simulink model "ModelMedusa"  (R2022b)
settings: Solver=FixedStepDiscrete  StartTime=0.0  StopTime=1  RelTol=1e-3  EnableMultiTasking=on
InitFcn:
  | % Initialize model
  | run(['ModelInit.m']);
  | 
  | % load library data
  | GainLibrary_data;
StartFcn:
  | % make sure all the simulated RTC requests are found
  | %RTC_SIM_OBJ.ValidateREQs();
model workspace (MAT data in the model file):
  PreampVolumeTable_Idx : Simulink.Signal (value not decoded)
  Range : Simulink.Signal (value not decoded)
  Table_Idx : Simulink.Signal (value not decoded)
undefined symbols (not defined in the file): Config, IFIR, Ifir, MedusaConfig, numAudioIn, Row, sys_defs, VLSConfig
libraries: TuneVar x16, FeaturePath x15, MedusaDelays x9, RTC x5, TOP x5, SampleRateConverter x4, dspindex x3, EdgePorts x2, MedusaCaeEnable x2, FIREven x2, VLSGains x2, dspsrcs4 x2
(part 2 of 2)

== system ModelMedusa/PreAmp/DecRate/Medusa5H1/MedusaHoligram/Medusa5H1 Part 4/On ==
  note: To fix the Headrest EQ link, FIR generic filter needs to work for multiple instances.
  HeadrestPremixOut : Inport
  NonHeadrestPremixOut : Inport  Port=2  OutDataTypeStr=single
  FRMixerOut : Inport  Port=3  OutDataTypeStr=single
  Action Port : ActionPort  ActionPortLabel=if(u1 > 0)
  DR Mix Matrix with Hybrid Holigram EQ : MedusaDRHoligramEQ/DR Holigram EQ  configStruct=config.HoligramEQConfig
  FR IIR Holigram EQ : MedusaFRHoligramEQ/FR Holigram EQ  configStruct=config.HoligramEQConfig
  Headrest Comp EQ : Subsystem  AncestorBlock=HeadrestCompEQ/Headrest Comp EQ  mask{configStruct=vlsConfigStruct.HeadrestCompEQConfig}
      mask prompts: configStruct "Config struct name:"
      mask init:
      | % Get block parameters from configStruct
      | fixedDelayLength = configStruct.fixedDelayLength;
      | IIR = configStruct.DRIIR;
      | variantFIR = configStruct.variantFIR;
      | variantIIR = configStruct.variantIIR;
      | firLength = configStruct.firLength;
      | frameSize = configStruct.frameSize;
      | numEQlink = configStruct.numEQlink;
      | numInput = configStruct.numInput;
      | 
      | % Get block default values
      | firCoeffsDefault = configStruct.firCoeffsDefault;
      | 
      | % Set implementation type for FIR
      | firBlockPath = MaskUtil.SubBlockName(gcbh, 'FIR');
      | firBlockHandle = getSimulinkBlockHandle(firBlockPath);
      | if -1 ~= firBlockHandle
      |     set_param(firBlockHandle, 'variantSelect', variantFIR);
      |     if variantFIR == 1 % Set two extras block params for Accel implementation
      |         set_param(firBlockHandle, 'numIn', num2str(numInput));
      |         set_param(firBlockHandle, 'frameSize', num2str(frameSize));
      |     end
      | end
      | 
      | iirBlockPath = MaskUtil.SubBlockName(gcbh, 'IIR');
      | iirBlockHandle = getSimulinkBlockHandle(iirBlockPath);
      | if -1 ~= iirBlockHandle
      |     set_param(iirBlockHandle, 'variantSelect', variantIIR);
      |     if variantIIR == 1 % Set two extras block params for Accel implementation
      |         set_param(iirBlockHandle, 'numChannels', num2str(numEQlink));
      |         set_param(iirBlockHandle, 'frameSize', num2str(frameSize));
      |     end
      | end
      settings: LibrarySourceBlock=HeadrestCompEQ/Headrest Comp EQ
  Matrix Concatenate : Concatenate  Mode=Multidimensional array  ConcatenateDimension=2
  DROut : Outport  VectorParamsAs1DForOutWhenUnconnected=off
  FROut : Outport  Port=2  VectorParamsAs1DForOutWhenUnconnected=off
  wires:
  FR IIR Holigram EQ/1 -> FROut/1
  Matrix Concatenate/1 -> DROut/1
  Headrest Comp EQ/1(Components Out) -> Matrix Concatenate/2
  DR Mix Matrix with Hybrid Holigram EQ/1 -> Matrix Concatenate/1
  FRMixerOut/1 -> FR IIR Holigram EQ/1
  NonHeadrestPremixOut/1 -> DR Mix Matrix with Hybrid Holigram EQ/1
  HeadrestPremixOut/1 -> Headrest Comp EQ/1(Components In)

== system ModelMedusa/PreAmp/DecRate/Medusa5H1/MedusaHoligram/Medusa5H1 Part 5/Speaker Delay Tune ==
  Output Delay Translation with Headrest : MedusaDelays/HeadrestOutputDelayTranslation  Config=[]
  TOP3 : TOP/TOP  TriggerInit=[645 305 895 365]  TopName=FRSpeakerDelay  DataType=int32  BankNumber=0  PreOverlay=false  PostOverlay=false  Role=Automatic
      settings: SourceProductName=Bose Talaria
  TOP5 : TOP/TOP  TriggerInit=[645 155 895 215]  TopName=DRSpeakerDelay  DataType=int32  BankNumber=0  PreOverlay=false  PostOverlay=false  Role=Automatic
      settings: SourceProductName=Bose Talaria
  Tune Variable : TuneVar/TuneVar  TuneName=HeadrestDrvSpeakerDelaySamples  SpecifyMaxSize=off  VariableDim=1 (Row)  MaxSize=[1 1]  TunabilityNumber=1  MinValue=[]  MaxValue=[]  TriggerInit=[20 195 245 245]  MaskValue=[0]
      settings: SourceProductName=Bose Talaria
  Tune Variable1 : TuneVar/TuneVar  TuneName=NonHeadrestSpeakerDelaySamples  SpecifyMaxSize=off  VariableDim=1 (Row)  MaxSize=[1 1]  TunabilityNumber=1  MinValue=[]  MaxValue=[]  TriggerInit=[20 120 245 170]  MaskValue=HRDelayConfig.DRNonHRDelay
      settings: SourceProductName=Bose Talaria
  Tune Variable4 : TuneVar/TuneVar  TuneName=HeadrestPaxSpeakerDelaySamples  SpecifyMaxSize=off  VariableDim=1 (Row)  MaxSize=[1 1]  TunabilityNumber=1  MinValue=[]  MaxValue=[]  TriggerInit=[20 270 245 320]  MaskValue=[0]
      settings: SourceProductName=Bose Talaria
  Tune Variable5 : TuneVar/TuneVar  TuneName=FRHoligramDelaySamples  SpecifyMaxSize=off  VariableDim=1 (Row)  MaxSize=[]  TunabilityNumber=1  MinValue=[]  MaxValue=[]  TriggerInit=[20 345 245 395]  MaskValue=HRDelayConfig.FRSpkrDelay
      settings: SourceProductName=Bose Talaria
  DRSpeakerDelay : Outport
  FRSpeakerDelay : Outport  Port=2
  wires:
  Output Delay Translation with Headrest/2 -> TOP3/1
  Output Delay Translation with Headrest/1 -> TOP5/1
  Tune Variable5/1 -> Output Delay Translation with Headrest/4  "FRHoligramDelaySamples"
  Tune Variable4/1 -> Output Delay Translation with Headrest/3  "HeadrestPaxSpeakerDelaySamples"
  Tune Variable/1 -> Output Delay Translation with Headrest/2  "HeadrestDrvSpeakerDelaySamples"
  Tune Variable1/1 -> Output Delay Translation with Headrest/1  "NonHeadrestSpeakerDelaySamples"
  TOP3/1 -> FRSpeakerDelay/1  "FRSpeakerDelay"
  TOP5/1 -> DRSpeakerDelay/1  "DRSpeakerDelay"

== system ModelMedusa/PreAmp/DecRate/Medusa5H1/MedusaHoligram/Medusa5H1 Part 1/CAE Treble Boost/Audio Passthrough ==
  AudioIn : Inport
  Constant : Constant  Value=0  OutDataTypeStr=int32  SampleTime=-1
  Constant3 : Constant  Value=0  OutDataTypeStr=int32  SampleTime=-1
  Target StateVar : StateVar/TargetStateVar  TriggerInit=[235 166 375 234]  TspName=DummyState  StateName=DummyState  UseSameName=on  IfdefMacro=[]
      settings: SourceProductName=Bose Talaria
  Terminator : Terminator
  TuneTOP : TuneVar/TuneTOP  TriggerInit=[50 262 220 318]  TopName=DummyTune  TuneName=DummyTune  DataType=single  TunabilityNumber=1  MinValue=[]  MaxValue=[]  BankNumber=0  PreOverlay=false  PostOverlay=false  UseSameName=on  MaskValue=[1]
      settings: SourceProductName=Bose Talaria
  Out : Outport
  CAEEnable : Outport  Port=2
  wires:
  Constant3/1 -> CAEEnable/1
  Constant/1 -> Target StateVar/1
  TuneTOP/1 -> Terminator/1
  AudioIn/1 -> Out/1

== system ModelMedusa/PreAmp/DecRate/Medusa5H1/MedusaHoligram/Medusa5H1 Part 1/CAE Treble Boost/CAE Treble Boost  ==
  AudioIn : Inport
  CAE Enable : MedusaCaeEnable/MedusaCaeEnable  Config=Config.CaeEnable  MaskMessageName=CAEEnable
  Treble Boost : TrebleBoost/TrebleBoostStereo  Config=Config.TrebleBoost
  Tune Variable4 : TuneVar/TuneVar  Description=|  TuneName=SurroundOn  SpecifyMaxSize=off  VariableDim=1 (Row)  MaxSize=[1 1]  TunabilityNumber=1  MinValue=[]  MaxValue=[]  TriggerInit=[-50 35 120 85]  MaskValue=2
      | General surround control parameter
      | STEREO_MODE = 0
      | SURROUND_PASSTHRU_MODE = 1
      | MEDUSA_2_CHANNEL_MODE = 2
      | MEDUSA_5_1_MODE = 3
      settings: SourceProductName=Bose Talaria
  Out : Outport
  CAEEnable : Outport  Port=2
  wires:
  Treble Boost/1 -> Out/1
  AudioIn/1 -> Treble Boost/1
  Tune Variable4/1 -> Treble Boost/2  "SurroundOn"
  CAE Enable/1 -> CAEEnable/1, Treble Boost/3

== system ModelMedusa/PreAmp/DecRate/Medusa5H1/MedusaHoligram/Medusa5H1 Part 1/Medusa Band Split Stereo/Interpolated Filter ==
  AudioIn : Inport
  Data Store Memory : DataStoreMemory  DataStoreName=states  ReadBeforeWriteMsg=warning  WriteAfterWriteMsg=warning  WriteAfterReadMsg=warning  InitialValue=zeros(size(coeffsFlip,1)*I,numChannels)  ShowAdditionalParam=off  OutDataTypeStr=single
  ifir : MATLAB Function  TreatAsAtomicUnit=on
  AudioOut : Outport  VectorParamsAs1DForOutWhenUnconnected=off
  wires:
  ifir/1(audioOut) -> AudioOut/1
  AudioIn/1 -> ifir/1(audioIn)

== system ModelMedusa/PreAmp/DecRate/Medusa5H1/MedusaHoligram/Medusa5H1 Part 3/On/Delay Tuning ==
  Delay Translation : MedusaDelays/MedusaAlignmentDelayTranslation  Config=Config.AlignmentDelayTranslation
  Tune Variable : TuneVar/TuneVar  TuneName=WiggleFilterDelayDecRateSamples1  SpecifyMaxSize=off  VariableDim=1 (Row)  MaxSize=[1 1]  TunabilityNumber=1  MinValue=[]  MaxValue=[]  TriggerInit=[-115 25 55 75]  MaskValue=Config.AlignmentDelayTranslation.DefaultTuning.DeciRateWiggleDelay
      settings: SourceProductName=Bose Talaria
  Tune Variable1 : TuneVar/TuneVar  TuneName=NEARWiggleFilterDelayDecRateSamples1  SpecifyMaxSize=off  VariableDim=1 (Row)  MaxSize=[1 1]  TunabilityNumber=1  MinValue=[]  MaxValue=[]  TriggerInit=[-115 87 55 133]  MaskValue=Config.AlignmentDelayTranslation.DefaultTuning.DeciRateNearWiggleDelay
      settings: SourceProductName=Bose Talaria
  Out1 : Outport
  Out2 : Outport  Port=2
  Out3 : Outport  Port=3
  wires:
  Tune Variable1/1 -> Delay Translation/2  "NEARWiggleFilterDelayDecRateSamples1"
  Delay Translation/3 -> Out3/1
  Delay Translation/1 -> Out1/1
  Delay Translation/2 -> Out2/1
  Tune Variable/1 -> Delay Translation/1  "WiggleFilterDelayDecRateSamples1"

== system ModelMedusa/PreAmp/DecRate/Medusa5H1/MedusaHoligram/Medusa5H1 Part 3/On/Expand Tail Components ==
  Tail Comps : Inport
  Constant : Constant  Value=[0 1 2 3]  OutDataTypeStr=single  SampleTime=-1
  Tail Component EQ : PooliirLib/PooliirwithNonTrivialTranslations  maxNumStages=tailCompEQ.maxNumStages  numStages=tailCompEQ.numStages  sosCoefficients=tailCompEQ.coeffs  FeatureName=tailCompEQ
  TuneTOP : TuneVar/TuneTOP  TriggerInit=[265 167 435 223]  TopName=WiggleFilter  TuneName=WiggleFilter  DataType=single  TunabilityNumber=1  MinValue=[]  MaxValue=[]  BankNumber=0  PreOverlay=false  PostOverlay=false  UseSameName=on  MaskValue=config.wiggleFilterDefault
      settings: SourceProductName=Bose Talaria
  Wiggle Filters : FIREven/FIR Even  variantSelect=Hexagon
      settings: SourceProductName=Bose Blocklib
  Wiggle Comps : Outport  VectorParamsAs1DForOutWhenUnconnected=off
  wires:
  Tail Comps/1 -> Wiggle Filters/1  "Ltail, Rtail, Ltail, Rtail"
  Tail Component EQ/1 -> Wiggle Comps/1
  Constant/1 -> Wiggle Filters/3
  TuneTOP/1 -> [wiggleFilter]
  Wiggle Filters/1 -> Tail Component EQ/1  "Lftail, Rftail, Lrtail, Rrtail"
  [wiggleFilter] -> Wiggle Filters/2

== system ModelMedusa/PreAmp/DecRate/Medusa5H1/MedusaHoligram/Medusa5H1 Part 3/On/Full-rate Mixer ==
  Upmix In : Inport
  CAE Control : Inport  Port=2
  Full-Rate Mixer with CAE & Fade Ramper : MedusaFullRateMixer/Full-Rate Mixer with CAE & Fade Ramper  MedusaFRMConfig=config.FRMConfig  MedusaFRMTune=config.FRMTune
  Out1 : Outport
  tag scope: NTFDone2=global
  wires:
  CAE Control/1 -> Full-Rate Mixer with CAE & Fade Ramper/9
  [SLC_On] -> Full-Rate Mixer with CAE & Fade Ramper/5
  [NTFCheck2] -> Full-Rate Mixer with CAE & Fade Ramper/8
  [BackFadeGain] -> Full-Rate Mixer with CAE & Fade Ramper/3
  [SurroundInfo] -> Full-Rate Mixer with CAE & Fade Ramper/7
  [SLCTrigger2] -> Full-Rate Mixer with CAE & Fade Ramper/6
  Full-Rate Mixer with CAE & Fade Ramper/2 -> [NTFDone2]
  [SLCReset2] -> Full-Rate Mixer with CAE & Fade Ramper/4
  [FrontFadeGain] -> Full-Rate Mixer with CAE & Fade Ramper/2
  Full-Rate Mixer with CAE & Fade Ramper/1 -> Out1/1
  Upmix In/1 -> Full-Rate Mixer with CAE & Fade Ramper/1

== system ModelMedusa/PreAmp/DecRate/Medusa5H1/MedusaHoligram/Medusa5H1 Part 3/On/Premix ==
  Bass In : Inport
  Upmix In : Inport  Port=2
  Wiggle In : Inport  Port=3
  CAE Control : Inport  Port=4
  Premix with Mono-Surround & CAE with Fade Ramper : MedusaPremix/PremixWithMonoSurroundAndCaeWithFadeRamper  MedusaPremixConfig=config.PremixConfig  MedusaPremixTune=config.PremixTune  MSConfig=config.MSConfig
  Out1 : Outport
  tag scope: NTFDone1=global
  wires:
  [SLC_On] -> Premix with Mono-Surround & CAE with Fade Ramper/7
  CAE Control/1 -> Premix with Mono-Surround & CAE with Fade Ramper/11
  Premix with Mono-Surround & CAE with Fade Ramper/1 -> Out1/1
  Premix with Mono-Surround & CAE with Fade Ramper/2 -> [NTFDone1]
  Upmix In/1 -> Premix with Mono-Surround & CAE with Fade Ramper/2
  Wiggle In/1 -> Premix with Mono-Surround & CAE with Fade Ramper/3
  [BackFadeGain] -> Premix with Mono-Surround & CAE with Fade Ramper/5
  [NTFCheck1] -> Premix with Mono-Surround & CAE with Fade Ramper/10
  [SLCReset1] -> Premix with Mono-Surround & CAE with Fade Ramper/6
  [SLCTrigger1] -> Premix with Mono-Surround & CAE with Fade Ramper/8
  [FrontFadeGain] -> Premix with Mono-Surround & CAE with Fade Ramper/4
  [SurroundInfo] -> Premix with Mono-Surround & CAE with Fade Ramper/9
  Bass In/1 -> Premix with Mono-Surround & CAE with Fade Ramper/1

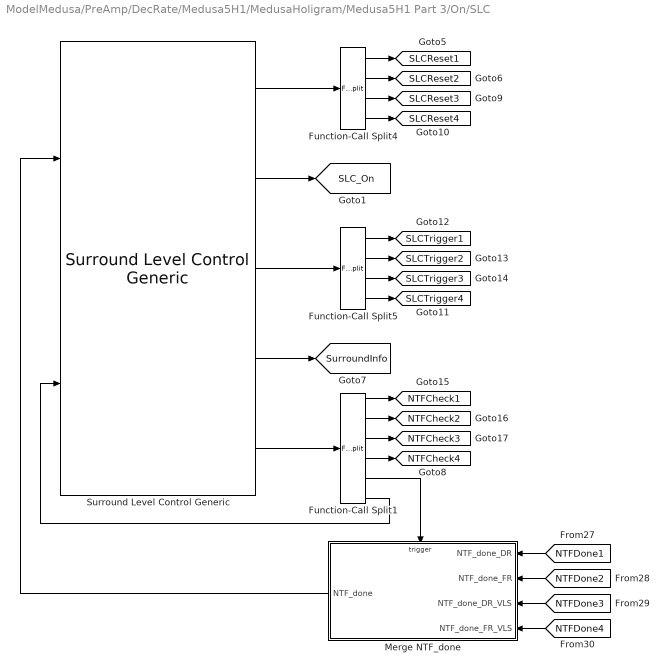
== system ModelMedusa/PreAmp/DecRate/Medusa5H1/MedusaHoligram/Medusa5H1 Part 3/On/SLC ==
  Function-Call Split1 : FunctionCallSplit  IconShape=distinctive  NumOutputPorts=6  OutputPortLayout=default
  Function-Call Split4 : FunctionCallSplit  IconShape=distinctive  NumOutputPorts=4  OutputPortLayout=default
  Function-Call Split5 : FunctionCallSplit  IconShape=distinctive  NumOutputPorts=4  OutputPortLayout=default
  Merge NTF_done : Subsystem
  Surround Level Control Generic : MedusaSurroundLevelControl/Surround Level Control Generic  SurroundConfig=config.SurroundConfig
  tag scope: NTFCheck1=global, NTFCheck2=global, NTFCheck3=global, NTFCheck4=global, SLCReset1=global, SLCReset2=global, SLCReset3=global, SLCReset4=global, SLCTrigger1=global, SLCTrigger2=global, SLCTrigger3=global, SLCTrigger4=global, SLC_On=global, SurroundInfo=global
  wires:
  Function-Call Split1/6 -> Surround Level Control Generic/2
  Surround Level Control Generic/2 -> [SLC_On]
  Surround Level Control Generic/5 -> Function-Call Split1/1
  Merge NTF_done/1(NTF_done) -> Surround Level Control Generic/1
  [NTFDone3] -> Merge NTF_done/3(NTF_done_DR_VLS)
  Function-Call Split4/4 -> [SLCReset4]
  Function-Call Split5/3 -> [SLCTrigger3]
  Function-Call Split5/1 -> [SLCTrigger1]
  Surround Level Control Generic/3 -> Function-Call Split5/1
  Surround Level Control Generic/4 -> [SurroundInfo]
  Function-Call Split4/1 -> [SLCReset1]
  Function-Call Split5/4 -> [SLCTrigger4]
  Function-Call Split4/3 -> [SLCReset3]
  [NTFDone4] -> Merge NTF_done/4(NTF_done_FR_VLS)
  Function-Call Split1/5 -> Merge NTF_done/Trigger
  Function-Call Split4/2 -> [SLCReset2]
  [NTFDone2] -> Merge NTF_done/2(NTF_done_FR)
  Function-Call Split1/4 -> [NTFCheck4]
  Function-Call Split5/2 -> [SLCTrigger2]
  Function-Call Split1/2 -> [NTFCheck2]
  Function-Call Split1/1 -> [NTFCheck1]
  [NTFDone1] -> Merge NTF_done/1(NTF_done_DR)
  Surround Level Control Generic/1 -> Function-Call Split4/1
  Function-Call Split1/3 -> [NTFCheck3]

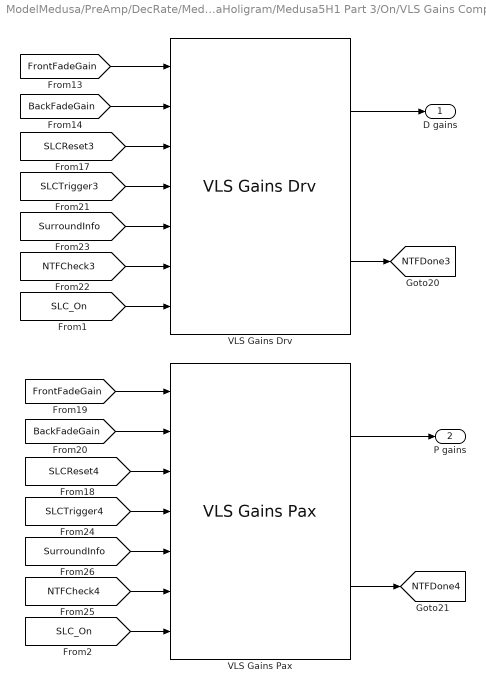
== system ModelMedusa/PreAmp/DecRate/Medusa5H1/MedusaHoligram/Medusa5H1 Part 3/On/VLS Gains Computation ==
  VLS Gains Drv : VLSGains/VLS Gains Drv  configStruct=vlsConfigStruct.VLSGainsConfig  tuneStruct=vlsConfigStruct.VLSGainsTune  FeatureName=VLSDrvGains
  VLS Gains Pax : VLSGains/VLS Gains Pax  configStruct=vlsConfigStruct.VLSGainsConfig  tuneStruct=vlsConfigStruct.VLSGainsTune  FeatureName=VLSPaxGains
  D gains : Outport
  P gains : Outport  Port=2
  tag scope: NTFDone3=global, NTFDone4=global
  wires:
  [SLC_On] -> VLS Gains Pax/7
  [SLC_On] -> VLS Gains Drv/7
  VLS Gains Pax/1 -> P gains/1
  VLS Gains Drv/1 -> D gains/1
  [FrontFadeGain] -> VLS Gains Drv/1
  [SLCReset4] -> VLS Gains Pax/3
  [SLCTrigger4] -> VLS Gains Pax/4
  [FrontFadeGain] -> VLS Gains Pax/1
  [SurroundInfo] -> VLS Gains Pax/5
  [NTFCheck4] -> VLS Gains Pax/6
  [BackFadeGain] -> VLS Gains Drv/2
  [SLCTrigger3] -> VLS Gains Drv/4
  VLS Gains Drv/2 -> [NTFDone3]
  VLS Gains Pax/2 -> [NTFDone4]
  [SurroundInfo] -> VLS Gains Drv/5
  [BackFadeGain] -> VLS Gains Pax/2
  [SLCReset3] -> VLS Gains Drv/3
  [NTFCheck3] -> VLS Gains Drv/6

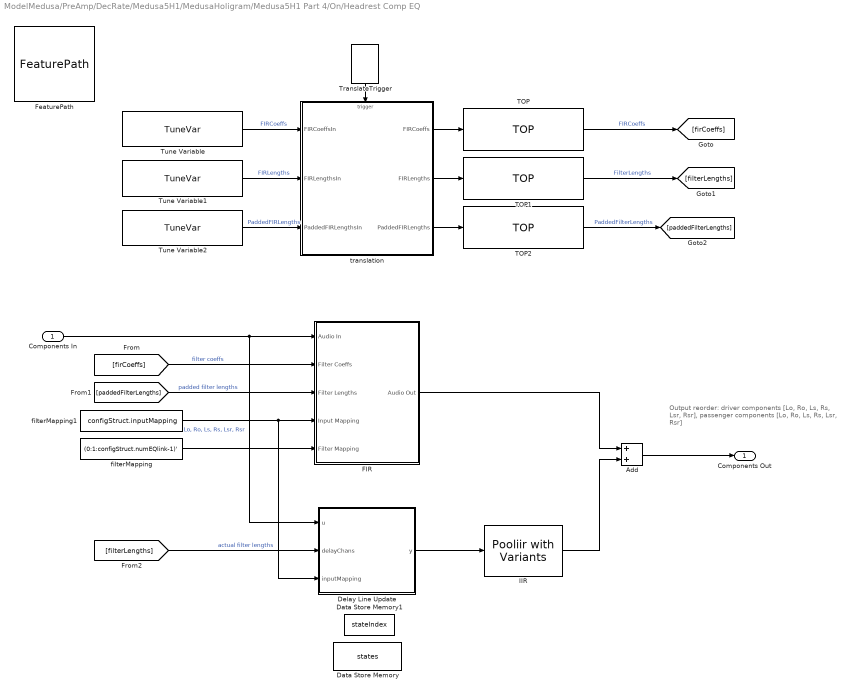
== system ModelMedusa/PreAmp/DecRate/Medusa5H1/MedusaHoligram/Medusa5H1 Part 4/On/Headrest Comp EQ ==
  note: Output reorder:
      | driver components [Lo, Ro, Ls, Rs, Lsr, Rsr],
      | passenger components [Lo, Ro, Ls, Rs, Lsr, Rsr]
  Components In : Inport
  Add : Sum  Priority=2
  Data Store Memory : DataStoreMemory  DataStoreName=states  ReadBeforeWriteMsg=warning  WriteAfterWriteMsg=warning  WriteAfterReadMsg=warning  InitialValue=zeros(fixedDelayLength, numInput)  ShowAdditionalParam=off  OutDataTypeStr=single
  Data Store Memory1 : DataStoreMemory  DataStoreName=stateIndex  ReadBeforeWriteMsg=warning  WriteAfterWriteMsg=warning  WriteAfterReadMsg=warning  ShowAdditionalParam=off  OutDataTypeStr=int32
  Delay Line Update : MATLAB Function  TreatAsAtomicUnit=on
  FIR : Subsystem  AncestorBlock=FIRGeneric/Generic FIR  mask(FIR Generic){variantSelect=Hexagon, stateBufferSize=configStruct.totalBufferSize, numOut=configStruct.numEQlink, frameSize=0, numIn=0}
      mask prompts: variantSelect "Implementation:"; stateBufferSize "State buffer size:"; numOut "Number of outputs:"; frameSize "Frame size:"; numIn "Number of inputs:"
      mask help:
      | Generic FIR is a configurable multi-channel FIR filter that supports one or more channels.  Different filter coefficients and number of coefficients can be used for each channel filter.  There can be fewer inputs than outputs, with some inputs routed to more than one output filter.   Identical filter configurations can also be used for multiple output filters.  The Generic FIR model supports three different implementations, selectable from the model mask:
      |
      | (i)  Core: FIR filters executing on core with target specific CRL support
      | (ii) Accel: FIR filters executing on IIR hardware accelerator, offloading MIPS usage from core
      | (iii) Hexagon: FIR filters executing on Hexagon DSP
      | (iv) Generic: FIR filters executing on core without CRL support
      |
      | NOTE: The Generic FIR codeWorkMemory buffer should always be mapped to L1 memory or core MIPS usage will increase.
      |
      | For more information, please see 'Help'.
      mask init:
      | % Create alias for code work memory buffer for each instance of model
      | FirGenericMask(gcbh, variantSelect);
      | 
      | % There are three implementation types:
      | % Type    Value  Description
      | % CORE    1      Optimized assembly running on core
      | % ACCEL   2      Computing offloaded to accelerator peripheral
      | % HEXAGON 3      Optimized C/assembly code running on Hexagon DSP
      | % GENERIC 4      Generic implementation for other targets without CRL
      | 
      | if variantSelect == 1
      |     % 6 variable size arrays (for input, coeffs, states, 
      |     % stateSharingEnabled, taps array per output channel,
      |     % and mapped audio input offsets) 
      |     % + 10 struct members
      |     codeWorkMemorySize = numOut * 6 + 10;  % words
      |     
      | elseif variantSelect == 2
      |     % Accelerator CRL code work memory size is equal to:
      |     %             sizeof(accelWorkMemory_t) + variableDataSize;
      |     % with variable data size dependent on number inputs, number outputs
      |     % and frame size.  NOTE: this must be updated to match the CRL code
      |     % if any changes are made to the accelWorkMemory_t structure.
      |     codeWorkMemorySize = 156 + (24 + numIn*48 + numOut*40);  % bytes
      |     codeWorkMemorySize = codeWorkMemorySize / 4;  % words (single)
      | 
      | elseif variantSelect == 3    
      |     codeWorkMemorySize = 156 + (24 + numIn*8 + numOut*(80 + 4*frameSize));  % bytes
      |     codeWorkMemorySize = codeWorkMemorySize / 4;  % words (single)
      |     
      | else
      |     % This is not used if there is no CRL
      |     codeWorkMemorySize = 1;
      | end
      settings: LibrarySourceBlock=FIRGeneric/Generic FIR
      mask Help:
      | Generic multi-channel FIR block supports multiple inputs, outputs and coefficient sets. Some inputs may drive multiple outputs, and this input sharing is specified by an input mapping per output. Some filters may be shared among multiple outputs, and this filter sharing is specified by a filter mapping per output. Input sharing assumes all filters sharing the same input have the same length to support state buffer sharing.
      | 
      | <b>Input signals: </b>
      | u: input channels [frame size x number of inputs]
      | coeffs: coefficient sets [total sum of filter lengths x 1]
      | filterLengths: array of filter lengths [number of filters x 1]
      | inputMapping: zero-based input mapping for each output [number of outputs x 1]
      | filterMapping:  zero-based filter mapping for each output [number of outputs x 1]
      | 
      | <b>Output signals: </b>
      | y: output channels [frame size x number of outputs]
      | 
      | <b>Mask parameters: </b>
      | Implementation: Core/Accel /Generic
      | State buffer size: total size of state buffer [total state buffer size x 1]
      | Number of outputs
      | Frame size
      | Number of inputs
      mask TypeOptions variantSelect: Core | Accel | Hexagon | Generic
      mask Callback variantSelect:
      | % Get the mask parameter value
      | maskStr = get_param(gcb,'variantSelect');
      | 
      | % Check the value of 'variantSelect'
      | if (~strcmp(maskStr,"Accel"))
      |     % Turn the visibility of 'frameSize' and 'numChannels' OFF
      |     set_param(gcb,'MaskVisibilities',{'on';'on';'on';'off';'off'});
      | else
      |     % "Accel": Set the visibility of all parameters to ON
      |     set_param(gcb,'MaskVisibilities',{'on';'on';'on';'on';'on'});
      | end
  FeaturePath : FeaturePath/FeaturePath  FeatureName=HeadrestCompEQ  IsGroup=off  GroupNumber=-1  IsModule=off  TriggerInit=[175 204 290 311]
      settings: SourceProductName=Bose Talaria
  IIR : PooliirAccel/Pooliir with Variants  variantSelect=Hexagon  maxNumStages=IIR.maxNumStages  numStages=IIR.numStages  sosCoefficients=IIR.coeffs  frameSize=0  numChannels=0  FeatureName=IIR
  TOP : TOP/TOP  TriggerInit=[815 320 985 380]  TopName=FIRCoeffs  DataType=single  BankNumber=1  PreOverlay=false  PostOverlay=false  Role=Automatic
      settings: SourceProductName=Bose Talaria
  TOP1 : TOP/TOP  TriggerInit=[815 390 985 450]  TopName=FilterLengths  DataType=uint32  BankNumber=0  PreOverlay=false  PostOverlay=false  Role=Automatic
      settings: SourceProductName=Bose Talaria
  TOP2 : TOP/TOP  TriggerInit=[815 460 985 520]  TopName=PaddedFilterLengths  DataType=uint32  BankNumber=0  PreOverlay=false  PostOverlay=false  Role=Automatic
      settings: SourceProductName=Bose Talaria
  TranslateTrigger : TuneVar/TranslateTrigger  TriggerInit=[656 230 694 285]
      settings: SourceProductName=Bose Talaria
  Tune Variable : TuneVar/TuneVar  TuneName=FIRCoeffs  SpecifyMaxSize=off  VariableDim=1 (Row)  MaxSize=[firLength*numEQlink 1]  TunabilityNumber=1  MinValue=[]  MaxValue=[]  TriggerInit=[330 325 500 375]  MaskValue=firCoeffsDefault
      settings: SourceProductName=Bose Talaria
  Tune Variable1 : TuneVar/TuneVar  TuneName=FIRLengths  SpecifyMaxSize=off  VariableDim=1 (Row)  MaxSize=[1 1]  TunabilityNumber=1  MinValue=[]  MaxValue=[]  TriggerInit=[330 395 500 445]  MaskValue=firLength*ones(numEQlink,1)
      settings: SourceProductName=Bose Talaria
  Tune Variable2 : TuneVar/TuneVar  TuneName=PaddedFIRLengths  SpecifyMaxSize=off  VariableDim=1 (Row)  MaxSize=[1 1]  TunabilityNumber=1  MinValue=[]  MaxValue=[]  TriggerInit=[330 465 500 515]  MaskValue=firLength*ones(numEQlink,1)
      settings: SourceProductName=Bose Talaria
  filterMapping : Constant  Value=(0:1:configStruct.numEQlink-1)'  VectorParams1D=off  OutDataTypeStr=uint32
  filterMapping1 : Constant  Value=configStruct.inputMapping  VectorParams1D=off  OutDataTypeStr=uint32
  translation : MATLAB Function  TreatAsAtomicUnit=on
  Components Out : Outport  VectorParamsAs1DForOutWhenUnconnected=off
  wires:
  Add/1 -> Components Out/1
  [firCoeffs] -> FIR/2(Filter Coeffs)  "filter coeffs"
  FIR/1(Audio Out) -> Add/1
  translation/2(FIRLengths) -> TOP1/1
  IIR/1 -> Add/2
  Tune Variable1/1 -> translation/2(FIRLengthsIn)  "FIRLengths"
  TOP/1 -> [firCoeffs]  "FIRCoeffs"
  filterMapping/1 -> FIR/5(Filter Mapping)
  translation/1(FIRCoeffs) -> TOP/1
  Delay Line Update/1(y) -> IIR/1
  TranslateTrigger/1 -> translation/Trigger
  Tune Variable/1 -> translation/1(FIRCoeffsIn)  "FIRCoeffs"
  filterMapping1/1 -> FIR/4(Input Mapping), Delay Line Update/3(inputMapping)
  [paddedFilterLengths] -> FIR/3(Filter Lengths)  "padded filter lengths"
  TOP1/1 -> [filterLengths]  "FilterLengths"
  Components In/1 -> FIR/1(Audio In), Delay Line Update/1(u)  "Lo, Ro, Ls, Rs, Lsr, Rsr"
  Tune Variable2/1 -> translation/3(PaddedFIRLengthsIn)  "PaddedFIRLengths"
  TOP2/1 -> [paddedFilterLengths]  "PaddedFilterLengths"
  translation/3(PaddedFIRLengths) -> TOP2/1
  [filterLengths] -> Delay Line Update/2(delayChans)  "actual filter lengths"

== system ModelMedusa/PreAmp/DecRate/Medusa5H1/MedusaHoligram/Medusa5H1 Part 3/On/SLC/Merge NTF_done ==
  NTF_done_DR : Inport
  NTF_done_FR : Inport  Port=2
  NTF_done_DR_VLS : Inport  Port=3
  NTF_done_FR_VLS : Inport  Port=4
  Trigger : TriggerPort  TriggerType=function-call  VariantControl=Variant  PortDimensions=1
  AND : Logic  Inputs=4  IconShape=distinctive  AllPortsSameDT=off  OutDataTypeStr=boolean
  NTF_done : Outport  VectorParamsAs1DForOutWhenUnconnected=off
  wires:
  NTF_done_FR_VLS/1 -> AND/4
  NTF_done_DR_VLS/1 -> AND/3
  NTF_done_DR/1 -> AND/1
  NTF_done_FR/1 -> AND/2
  AND/1 -> NTF_done/1

== system ModelMedusa/PreAmp/DecRate/Medusa5H1/MedusaHoligram/Medusa5H1 Part 4/On/Headrest Comp EQ/FIR ==
  Audio In : Inport
  Filter Coeffs : Inport  Port=2
  Filter Lengths : Inport  Port=3
  Input Mapping : Inport  Port=4
  Filter Mapping : Inport  Port=5
  FIR generic init : MATLAB Function  TreatAsAtomicUnit=on  RTWFcnName=foo
  FeaturePath : FeaturePath/FeaturePath  FeatureName=FIR  IsGroup=off  GroupNumber=-1  IsModule=off  TriggerInit=[105 -141 220 -34]
      settings: SourceProductName=Bose Talaria
  ITC : Subsystem  mask(Bose Initialization Trigger Control){}
      mask help: This block emits a function trigger for logic intended to execute at subsystem initialization time. Make sure not to reference any "live" signals
      mask init:
      | CodeID = InitTriggerControlMask.DoInit(gcbh);
      | ok = true;
      mask Display:
      | % retrieve icon definition
      | [path,w,h] = InitTriggerControlMask.Icon();
      | 
      | % retrieve the block's pixel size
      | pos = get(gcbh,'position');
      | bw = pos(3) - pos(1);
      | bh = pos(4) - pos(2);
      | 
      | % draw  icon to the center left
      | xAdj = bw/2 - w/2;
      | yAdj = bh/2 - h/2 + 4;
      | for i=1:length(path)
      |     patch(path(i).x+xAdj, path(i).y+yAdj, path(i).rgb);
      | end
      | 
      | text(bw*0.5, bh*0.2, 'ITC', 'horizontalAlignment', 'center');
      | 
      | % show X on error
      | if (exist('ok','var') && ok)
      | 	patch(0,0,[1 1 1]);
      | 	patch(bw,bh,[1 1 1]);
      | else
      | 	tx=bw*0.03;
      | 	ty=bh*0.03;
      | 	patch([0 tx bw bw-tx], [ty 0 bh-ty bh], [1 0 0]);
      | 	patch([0 bw-tx bw tx], [bh-ty 0 ty bh], [1 0 0]);
      | end
  MATLAB Function : MATLAB Function  TreatAsAtomicUnit=on
  codeWorkMemory : DataStoreMemory  DataStoreName=codeWorkMemory  WriteAfterWriteMsg=warning  InitialValue=zeros(1,codeWorkMemorySize)  ShowAdditionalParam=off  OutDataTypeStr=uint32
  stateBuffer : DataStoreMemory  DataStoreName=states  ReadBeforeWriteMsg=warning  WriteAfterWriteMsg=warning  WriteAfterReadMsg=warning  InitialValue=zeros(stateBufferSize,1)  ShowAdditionalParam=off  OutDataTypeStr=single
  Audio Out : Outport  VectorParamsAs1DForOutWhenUnconnected=off
  wires:
  Audio In/1 -> MATLAB Function/1(u), FIR generic init/1(u)
  ITC/1(Out1) -> FIR generic init/Trigger
  MATLAB Function/1(y) -> Audio Out/1
  Filter Mapping/1 -> MATLAB Function/5(filterMapping), FIR generic init/5(filterMapping)
  Filter Coeffs/1 -> MATLAB Function/2(coeffs), FIR generic init/2(coeffs)
  Input Mapping/1 -> MATLAB Function/4(inputMapping), FIR generic init/4(inputMapping)
  Filter Lengths/1 -> MATLAB Function/3(filterLengths), FIR generic init/3(filterLengths)

== system ModelMedusa/PreAmp/DecRate/Medusa5H1/MedusaHoligram/Medusa5H1 Part 4/On/Headrest Comp EQ/FIR/ITC ==
  ITC1 : S-Function  FunctionName=InitTriggerControl  Parameters=CodeID, 0  SFunctionDeploymentMode=off  EnableBusSupport=off
  init : MATLAB Function  TreatAsAtomicUnit=on  RTWFcnName=InitTrigger_ModelMedusa_4079_595_209_62
      settings: RTWSystemCode=Nonreusable function
  Out1 : Outport  VectorParamsAs1DForOutWhenUnconnected=off
  wires:
  init/1(init()) -> Out1/1
  ITC1/1 -> init/Trigger

== matlab function ModelMedusa/PreAmp/DecRate/Medusa5H1/MedusaHoligram/Medusa5H1 Part 1/Medusa Band Split Stereo/Interpolated Filter/ifir ==
  data: audioIn input; coeffsFlip parameter; audioOut output; I parameter; states data_store_memory
function audioOut = ifir(audioIn, coeffsFlip, I)

% An interpolated FIR filter is an FIR filter with a sparse set of
% coefficients.  That is, the coefficients contain I-1 zeros between
% each point, so the effective length of  filter is len(input_coeffs) * I  
% The function support multiple channels, with each
% channel sharing the same set of filter coefficients.
% 
% p : coefficient set (non-zero coefficients)
% I : interpolation factor, I-1 zeros are inserted between each coefficient
% 
% NOTES: 
% The legacy IFIR block supported coefficient sets.  Currently
% this only supports one coefficient set. 
% The coefficients are stored flipped in time. The unflipped coeffs are
% passed to block mask, and the flipping is done in mask initialization.

% Initialize variables
[frameSize, numChannels] = size(audioIn);
[filterLength, ~] = size(coeffsFlip);

frameSize   = uint32(frameSize);
numChannels = uint32(numChannels);
filterLength = int32(filterLength);
activeCoeffSet = coder.const(uint32(zeros(1,numChannels)));

% State is a circular buffer that holds previous stateLen samples, 
% where state_index points to the last/oldest sample in the buffer, which 
% during processing will be overwritten by the current input sample.
global states;

persistent state_index;
if isempty(state_index)
    state_index = int32(0);
end

audioOut = IFIR(audioIn, frameSize, numChannels, states, filterLength, ...
                    state_index, coeffsFlip, activeCoeffSet, I);
                
end

function y = IFIR(audioIn, frameSize, numChannels, states2, filterLength, ...
                    state_index2, coeffsFlip, activeCoeffSet, I)
% If code gen'ing, generate warning if this is not replaced with IFIR.asm
%coder.replace('-warnifnoreplacement');

% We have to use a different state buffer and state index than the one 
% passed in.  Matlab value objects are passed by value, not by reference, 
% so the saving of states here does not work.  The state buffer and index 
% are still necessary to pass allocate in the calling function and pass 
% here in order to trigger CRL. This double buffering is annoying, however 
% only happens during simulation, not code generation. (taken from pooliir)
global states;
persistent state_index;
if isempty(state_index)
    state_index = int32(0);
end

y = coder.nullcopy(audioIn);
stateLen = filterLength * I;

for channel = 1:numChannels
    state = states(:,channel);
    stateIndex = state_index;
    coeffs = coeffsFlip(:,activeCoeffSet(channel)+1);
    
    for sample = 1:frameSize
        % overwrite oldest sample with the current input sample
        state(stateIndex+1) = audioIn(sample, channel);
        % go to the oldest sample (previously the 2nd oldest)
        stateIndex = stateIndex + I; 
        if (stateIndex >= stateLen)
            stateIndex = stateIndex - stateLen;
        end

        accum = single(0);
        for i = 1:filterLength
            accum = accum + (state(stateIndex+1) * coeffs(i));
            stateIndex = stateIndex + I; % skip zero coefficients
            if (stateIndex >= stateLen)
                    stateIndex = stateIndex - stateLen;
            end
        end
        y(sample, channel) = accum;

        % update stateIndex for next sample
        % because we subtract here state_index type is int32 not uint32
        stateIndex = stateIndex - (I-1);
        if (stateIndex < 0)
            stateIndex = stateIndex + stateLen;
        end
    end
 
    states(:, channel) = state;
end

state_index = stateIndex;

end

== matlab function ModelMedusa/NEAR/MATLAB Function ==
  data: u input; y output
function y = fcn(u)

y = u;

== matlab function ModelMedusa/PreAmp/Reset/MATLAB Function ==
  events: trigger input FUNCTION_CALL_EVENT
function fcn()

if coder.target('Rtw')
    coder.ceval('Model_Target_DRFDP_initialize');
    coder.ceval('Model_Target_FRFDP_initialize');
    coder.ceval('Model_Target_ExpandTailComponents_initialize');
    coder.ceval('Model_Target_TrebleandSurroundDelays_initialize');
    coder.ceval('Model_Target_Medusa5H1Part3_initialize');
    coder.ceval('Model_Target_Subsystem_initialize');
    
    coder.ceval('Model_Target_PreAmpPart1_Start');
    coder.ceval('Model_Target_SRCIn_Start');
%     coder.ceval('Model_Target_AudioPilot35_Start');
    coder.ceval('Model_Target_Medusa5H1Part1_Start');
    coder.ceval('Model_Target_Medusa5H1Part2_Start');
    coder.ceval('Model_Target_Medusa5H1Part3_Start');

    coder.ceval('Model_Target_PreAmpPart1_Init');
    coder.ceval('Model_Target_PreAmpPart2_Init');
%     coder.ceval('Model_Target_SRCIn_Init');
%     coder.ceval('Model_Target_SRCOut_Init');
%     coder.ceval('Model_Target_AudioPilot35_Init');
    coder.ceval('Model_Target_Medusa5H1Part1_Init');
    coder.ceval('Model_Target_Medusa5H1Part2_Init');
    coder.ceval('Model_Target_Medusa5H1Part3_Init');
end

== matlab function ModelMedusa/InputSelect/Reset/MATLAB Function ==
  events: trigger input FUNCTION_CALL_EVENT
function fcn()

if coder.target('Rtw')
    coder.ceval('Model_Target_InputSelect_Init');
end

== matlab function ModelMedusa/PreAmp/DecRate/Medusa5H1/MedusaHoligram/Medusa5H1 Part 4/On/Headrest Comp EQ/FIR/FIR generic init ==
  data: u input; coeffs input; filterLengths input; inputMapping input; filterMapping input; states data_store_memory; codeWorkMemory data_store_memory; variantSelect parameter
  events: trigger input FUNCTION_CALL_EVENT
function fir_generic_init(u,coeffs, filterLengths, inputMapping, filterMapping, variantSelect)

% Generic FIR function to work with M inputs, N outputs and K filters
%
% Parameters:
%   u:              input channels [frame size x number of inputs]
%   coeffs:         coefficient sets [total filter lengths x 1]
%   filterLengths:  array of filter lengths [number of filters x 1]
%   inputMapping:   zero-based input mapping for each filter  [number of outputs x 1]
%   filterMapping:  zero-based filter mapping for each filter [number of outputs x 1]
%
% Global parameters:
%   states:         array of states [totalBufferSize x 1]
%   codeWorkMemory: working memory set up during roommode reset/init CRL
%                   function call [codeWorkMemorySize x 1]

% Extract configuration information from inputs
[frame_size, num_inputs]  = size(u);
num_outputs = numel(inputMapping);

global states;
global codeWorkMemory;

% Get the work memory and states size
workMemorySize = numel(codeWorkMemory);
statesSize = numel(states);

% Set correct data types
filter_length = uint32(filterLengths);
numCoeffSets = uint32(numel(filter_length));
frame_size = uint32(frame_size);
num_outputs = uint32(num_outputs);
num_inputs = uint32(num_inputs);
workMemorySize = uint32(workMemorySize);
statesSize = uint32(statesSize);
    
% There are three implementation types:
% Type    Value   Description
% CORE    1       Optimized assembly running on core
% ACCEL   2       Computing offloaded to accelerator peripheral
% Hexagon 3       Optimized C code running on Hexagon DSP
% GENERIC 4       Generic implementation for other targets without CRL 
%
% NOTE: GENERIC implementation does not use codeWorkMemory, thus does not
% need any custom initialization.
if (variantSelect == 1)
    y = fir_core_init(u, coeffs, states, filter_length, inputMapping, filterMapping, frame_size, numCoeffSets, num_inputs, num_outputs, codeWorkMemory);
    
    % NOTE: The CRL mechanism requires an output for the function call,
    % and appears to be optimized out if that return value isn't used. 
    % This is a dummy operation to make sure CRL ends up in generated code
    codeWorkMemory(1) = y; 
elseif (variantSelect == 2)
    y = fir_accelerator_init(u, coeffs, states, statesSize, filter_length, inputMapping, filterMapping, frame_size, ...
                             numCoeffSets, num_inputs, num_outputs, codeWorkMemory, workMemorySize);

    % NOTE: The CRL mechanism requires an output for the function call,
    % and appears to be optimized out if that return value isn't used. 
    % This is a dummy operation to make sure CRL ends up in generated code
    codeWorkMemory(1) = y; 
elseif (variantSelect == 3)
    y = fir_hexagon_init(u, coeffs, states, filter_length, inputMapping, filterMapping, frame_size, numCoeffSets, num_inputs, num_outputs, codeWorkMemory);
    
    % NOTE: The CRL mechanism requires an output for the function call,
    % and appears to be optimized out if that return value isn't used. 
    % This is a dummy operation to make sure CRL ends up in generated code
    codeWorkMemory(1) = y;

end

end


function y = fir_accelerator_init(u, coeffs, states, statesSize, filterLengths, inputMapping, filterMapping,...
                                  frameSize, numCoeffSets, numInputs, numOutputs, workMemory,...
                                  workMemorySize)                         
% If target == codegen, error out if no CRL found
coder.replace('-errorifnoreplacement');

% No init simulation code, but need to do something to ensure CRL does not
% get optimized out
y = workMemory(1) + 1;

end

function y = fir_core_init(u, coeffs, states, filterLengths, inputMapping, filterMapping,...
                             frameSize, numCoeffSets, numInputs, numOutputs, workMemory)
% If target == codegen, error out if no CRL found
coder.replace('-errorifnoreplacement');

% No init simulation code, but need to do something to ensure CRL does not
% get optimized out
y = workMemory(1) + 1;

end

function y = fir_hexagon_init(u, coeffs, states, filterLengths, inputMapping, filterMapping,...
                             frameSize, numCoeffSets, numInputs, numOutputs, workMemory)
% If target == codegen, error out if no CRL found
coder.replace('-errorifnoreplacement');

% No init simulation code, but need to do something to ensure CRL does not
% get optimized out
y = workMemory(1) + 1;

end

== matlab function ModelMedusa/PreAmp/DecRate/Medusa5H1/MedusaHoligram/Medusa5H1 Part 4/On/Headrest Comp EQ/FIR/ITC/init ==
  events: trigger input FUNCTION_CALL_EVENT; init output FUNCTION_CALL_EVENT
function init

init();

== matlab function ModelMedusa/PreAmp/DecRate/Medusa5H1/MedusaHoligram/Medusa5H1 Part 4/On/Headrest Comp EQ/FIR/MATLAB Function ==
  data: u input; y output; coeffs input; filterLengths input; inputMapping input; filterMapping input; states data_store_memory; variantSelect parameter; codeWorkMemory data_store_memory
function y = fir_generic(u, coeffs, filterLengths, inputMapping, filterMapping, variantSelect)
% Generic FIR function to work with M inputs, N outputs and K filters
%
% Parameters:
%   u:              input channels [frame size x number of inputs]
%   coeffs:         coefficient sets [total filter lengths x 1]
%   filterLengths:  array of filter lengths [number of filters x 1]
%   inputMapping:   zero-based input mapping for each filter  [number of outputs x 1]
%   filterMapping:  zero-based filter mapping for each filter [number of outputs x 1]
%
% Global parameters:
%   states:         array of states [totalBufferSize x 1]
%   codeWorkMemory: working memory set up during roommode reset/init CRL
%                   function call [codeWorkMemorySize x 1]

% Extract configuration information from inputs
[frame_size, num_inputs]  = size(u);
num_outputs = numel(inputMapping);

global states;
global codeWorkMemory;
    
% Set correct data types
filter_length = uint32(filterLengths);
frame_size = uint32(frame_size);
num_outputs = uint32(num_outputs);
num_inputs = uint32(num_inputs);

% Define one-frame delay buffer only for Accelerator simulation 
% Simulink will optimize this out for code generation
persistent delayedOut;
if isempty(delayedOut)
    delayedOut = single(zeros(frame_size, num_outputs));
end
    
% There are three implementation types:
% Type    Value   Description
% CORE    1       Optimized assembly running on SHARC+ core
% ACCEL   2       Computing offloaded to SHARC+ accelerator peripheral
% Hexagon 3       Optimizaed C code running on Hexagon DSP
% GENERIC 4       Generic implementation for other targets without CRL

variantSelect=4;
variantSelect

% Simulation
if(coder.target('MATLAB') || coder.target('Sfun')) 
    if (variantSelect == 2)
        % Manually insert one-frame delay in simulation to mimic 
        % Accelerator behavior
        y = delayedOut;
        delayedOut = fir_generic_simulation(u, coeffs, states, filter_length, inputMapping, ...
                filterMapping, frame_size, num_inputs, num_outputs);
    else
        y = fir_generic_simulation(u, coeffs, states, filter_length, inputMapping, ...
                filterMapping, frame_size, num_inputs, num_outputs);
    end

% Code generation
else 
    if (variantSelect == 1)
        y = fir_core_process(u, codeWorkMemory, num_outputs);
    elseif (variantSelect == 2)
        y = fir_accelerator_process(u, codeWorkMemory, num_outputs);
    elseif (variantSelect == 3)
        y = fir_hexagon_process(u, codeWorkMemory, num_outputs);        
    else
        y = fir_generic_simulation(u, coeffs, states, filter_length, inputMapping, ...
                filterMapping, frame_size, num_inputs, num_outputs);
    end  
end

end


%% CRL functions for code generation
function y = fir_core_process(u, workMemory, numOutputs)
% If target == codegen, error out if no CRL found
coder.replace('-errorifnoreplacement');
[frameSize, ~]  = size(u);
y = single(zeros(frameSize, numOutputs));
end

function y = fir_accelerator_process(u, workMemory, numOutputs)
% If target == codegen, error out if no CRL found
coder.replace('-errorifnoreplacement');
[frameSize, ~]  = size(u);
y = single(zeros(frameSize, numOutputs));
end

function y = fir_hexagon_process(u, workMemory, numOutputs)
% If target == codegen, error out if no CRL found
coder.replace('-errorifnoreplacement');
[frameSize, ~]  = size(u);
y = single(zeros(frameSize, numOutputs));
end

== matlab function ModelMedusa/PreAmp/DecRate/Medusa5H1/MedusaHoligram/Medusa5H1 Part 4/On/Headrest Comp EQ/Delay Line Update ==
  data: u input; y output; delayChans input; inputMapping input; states data_store_memory; stateIndex data_store_memory; fixedDelayLength parameter
function y = delayLineUpdate(u, delayChans, inputMapping, fixedDelayLength)

% Note: This block only reads 'states' to get the delayed samples. A
% separate function is responsible for writing to 'states' to update the 
% delay line Data Store Memory. Thus it is important to ensure all DSM  
% write happens before DSM read.
%
% This is different from pooldelay, as the delay for ALL channel is
% intentionally set to be the max amount to allow for 'double' sharing
% between FIR filter and delay buffer.

global states;
global stateIndex; 

numOutput = numel(delayChans);
[frameSize, numChannelIn] = size(u);
y = single(zeros(frameSize, numOutput));
delayChans = int32(delayChans);

% Write incoming input to delay line
writeIdx = stateIndex;
for sample = 1:frameSize
    for i = 1:numChannelIn
        states(writeIdx+1,i) = u(sample, i); % add 1 for Matlab indexing
    end
    writeIdx = circindex(writeIdx, int32(1), fixedDelayLength);
end
stateIndex = writeIdx;

% Read out values from delay line
for i = 1:numOutput
    inputIdx = inputMapping(i);  % which input to delay
    delay = delayChans(i);       % delay amount
    offset = - (delay + frameSize); % offset from start index
    readIdx = circindex(stateIndex, offset, fixedDelayLength);
    
    for sample = 1:frameSize
        y(sample, i) = states(readIdx+1, inputIdx+1); % add 1 for Matlab indexing
        readIdx = circindex(readIdx, int32(1), fixedDelayLength);
    end
end

== matlab function ModelMedusa/PreAmp/DecRate/Medusa5H1/MedusaHoligram/Medusa5H1 Part 4/On/Headrest Comp EQ/translation ==
  data: FIRCoeffs output; FIRCoeffsIn input; FIRLengths output; FIRLengthsIn input; PaddedFIRLengthsIn input; PaddedFIRLengths output
  events: trigger input FUNCTION_CALL_EVENT
function [FIRCoeffs, FIRLengths, PaddedFIRLengths] = fcn(FIRCoeffsIn, FIRLengthsIn, PaddedFIRLengthsIn)

FIRCoeffs = FIRCoeffsIn.Value;
FIRLengths = FIRLengthsIn.Value;
PaddedFIRLengths = PaddedFIRLengthsIn.Value;
